simulink model "arm_2dof"  (R2025b)
settings: Solver=ode45  StartTime=0.0  StopTime=10  MaxStep=0.01  RelTol=1e-6
settings Model: Creator=Krishang  LastModifiedBy=Krishang

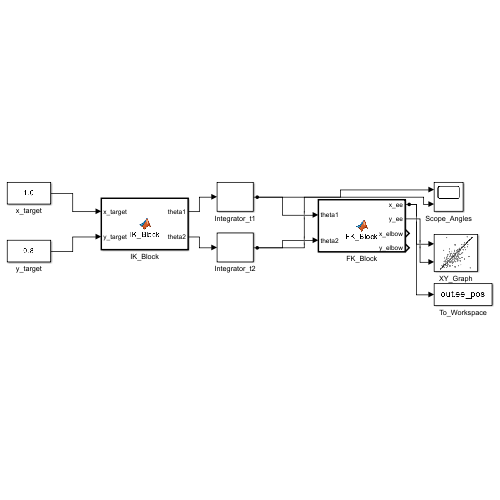
[thumbnail: Simulink's stored preview of the top-level diagram]
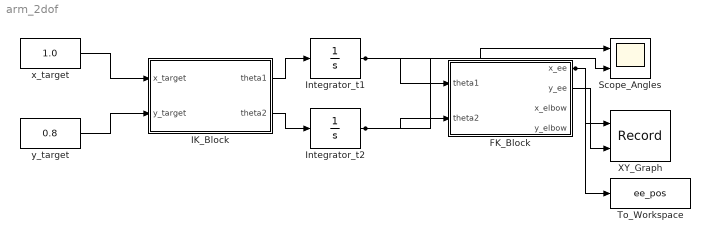
== system arm_2dof ==
  FK_Block : MATLAB Function  TreatAsAtomicUnit=on
  IK_Block : MATLAB Function  TreatAsAtomicUnit=on
  Integrator_t1 : Integrator
  Integrator_t2 : Integrator
  Scope_Angles : Scope  NumInputPorts=2
  To_Workspace : ToWorkspace  VariableName=ee_pos  SampleTime=-1
      settings: MaxDataPoints=10000
  XY_Graph : Record  NumPorts=2.0  FileSettingsInternal="{\"entries\":[{\"content\":{\"excelSettings\":{\"content\":{},\"type\":\"Streamout.ExcelSettings\"},\"parquetSettings\":{\"content\":{},\"type\":\"Streamout.ParquetSettings\"}},\"type\":\"Streamout.FileSettingStorage\",\"uuid\":\"\"}],\"packageUris\":[\"http:\\/\\/schema.mathworks.com\\/mf0\\/streamout_blocks\\/R2020a\"],\"version\":\"1.0\"}"  FrameSettings=[0, 0]  Layout=[1 1]  SignalsInternal="{\"entries\":[{\"content\":{\"signals\":[{\"content\":{\"blockPath\":[],\"dimensions\":[1],\"domain\":\"\",\"lineColor\":\"#a2142f\",\"plots\":[ 1 ],\"port\":1,\"signalID\":1,\"signalName\":\"XY Graph:1\"},\"type\":\"RecordBlkView.Signal\",\"uuid\":\"\"},{\"content\":{\"blockPath\":[],\"dimensions\":[1],\"domain\":\"\",\"lineColor\":\"#139fff\",\"plots\":[ 1 ],\"port\":2,\"signalID\":2,\"signalName\":\"XY Graph:2\"},\"type\":\"RecordBlkView.Signal\",\"uuid\":\"\"}]},\"type\":\"RecordBlkView.InputSignals\",\"uuid\":\"\"}],\"packageUris\":[\"http:\\/\\/schema.mathworks.com\\/mf0\\/streamout_blocks\\/R2020a\"],\"version\":\"1.0\"}"  VisualizationBindings="{\"xyplotplugin\":{\"info\":[{\"series\":[{\"bindingParametersList\":[{\"parameter\":\"X-Axis\",\"signalID\":1,\"signalName\":\"XY Graph:1\"},{\"parameter\":\"Y-Axis\",\"signalID\":2,\"signalName\":\"XY Graph:2\"}],\"seriesID\":0}],\"subplotID\":1}]}}"  CompatibilityTag=XY
  x_target : Constant  Value=1.0
  y_target : Constant  Value=0.8
  wires:
  x_target/1 -> IK_Block/1(x_target)
  y_target/1 -> IK_Block/2(y_target)
  IK_Block/1(theta1) -> Integrator_t1/1
  IK_Block/2(theta2) -> Integrator_t2/1
  Integrator_t1/1 -> FK_Block/1(theta1), Scope_Angles/1
  Integrator_t2/1 -> FK_Block/2(theta2), Scope_Angles/2
  FK_Block/1(x_ee) -> XY_Graph/1, To_Workspace/1
  FK_Block/2(y_ee) -> XY_Graph/2

== matlab function arm_2dof/FK_Block ==
  data: theta1 input; x_ee output; theta2 input; y_ee output; x_elbow output; y_elbow output
function [x_ee, y_ee, x_elbow, y_elbow] = FK_Block(theta1, theta2)
L1 = 1.0; L2 = 0.8;
x_elbow = L1 * cos(theta1);
y_elbow = L1 * sin(theta1);
x_ee    = x_elbow + L2 * cos(theta1 + theta2);
y_ee    = y_elbow + L2 * sin(theta1 + theta2);
end

== matlab function arm_2dof/IK_Block ==
  data: x_target input; theta1 output; y_target input; theta2 output
function [theta1, theta2] = IK_Block(x_target, y_target)
L1 = 1.0; L2 = 0.8;
r = sqrt(x_target^2 + y_target^2);
r_max = L1 + L2; r_min = abs(L1 - L2);
r_safe = max(r_min + 1e-6, min(r_max - 1e-6, r));
if r > 1e-9
    x_s = x_target * (r_safe / r);
    y_s = y_target * (r_safe / r);
else
    x_s = r_safe; y_s = 0;
end
c2 = (x_s^2 + y_s^2 - L1^2 - L2^2) / (2*L1*L2);
c2 = max(-1, min(1, c2));
s2 = sqrt(1 - c2^2);
theta2 = atan2(s2, c2);
alpha = atan2(y_s, x_s);
beta  = atan2(L2*sin(theta2), L1 + L2*cos(theta2));
theta1 = atan2(sin(alpha - beta), cos(alpha - beta));
end
